simulink model "ModelNonLinear"  (R2014b)
settings: Solver=ode45  StartTime=0.0  StopTime=5  FixedStep=0.01  RelTol=1e-3
values from neighbouring files (symbols this model uses):
  H1 = -(R4*Rs/R1) * 1/(R7+Rv2)    [InitModel.m]    (also in SystemModel.m)
  R6 = 100e3    (= 100000)    [InitModel.m]    (also in SystemModel.m; SystemModel_marco.m)
  rad2rpm = 60/(2*pi)    (= 9.54929658551)    [InitModel.m]    (also in SystemModel.m)
  Vdc = 30    [InitModel.m]    (also in SystemModel.m; SystemModel_marco.m)
undefined symbols (not defined in the file or in its folder): motor, sigbuilder_block
libraries: cstblocks x5, simulink x1
settings Model: Creator=Edoardo  LastModifiedBy=Edoardo

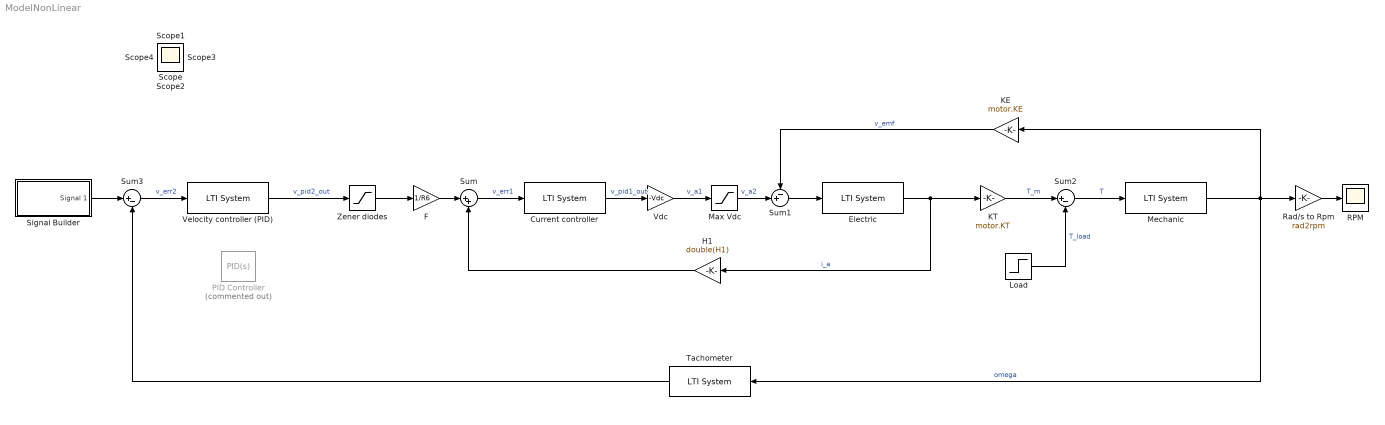
== system ModelNonLinear ==
  Current controller : cstblocks/LTI System  sys=C1  IC=[]
  Electric : cstblocks/LTI System  sys=G1  IC=[]
  F : Gain  Gain=1/R6
  H1 : Gain  Gain=double(H1)
  KE : Gain  Gain=motor.KE
  KT : Gain  Gain=motor.KT
  Load : Step  Time=2  After=0.02  SampleTime=0
  Max Vdc : Saturate  UpperLimit=30  LowerLimit=-30
  Mechanic : cstblocks/LTI System  sys=G2  IC=[]
  PID Controller : simulink/Continuous/PID Controller  Commented=on  Controller=PID  TimeDomain=Continuous-time  SampleTime=-1  IntegratorMethod=Forward Euler  FilterMethod=Forward Euler  Form=Parallel  P=9  I=18  D=0.001  N=100  InitialConditionSource=internal  InitialConditionForIntegrator=0  InitialConditionForFilter=0  ExternalReset=none  LimitOutput=off  UpperSaturationLimit=inf  LowerSaturationLimit=-inf  LinearizeAsGain=on  AntiWindupMode=none  Kb=1  TrackingMode=off  Kt=1  PParamMin=[]  PParamMax=[]  IParamMin=[]  IParamMax=[]  DParamMin=[]  DParamMax=[]  NParamMin=[]  NParamMax=[]  KbParamMin=[]  KbParamMax=[]  KtParamMin=[]  KtParamMax=[]  POutMin=[]  POutMax=[]  IOutMin=[]  IOutMax=[]  DOutMin=[]  DOutMax=[]  NOutMin=[]  NOutMax=[]  KbOutMin=[]  KbOutMax=[]  KtOutMin=[]  KtOutMax=[]  IntegratorOutMin=[]  IntegratorOutMax=[]  FilterOutMin=[]  FilterOutMax=[]  SumOutMin=[]  SumOutMax=[]  SumI1OutMin=[]  SumI1OutMax=[]  SumI2OutMin=[]  SumI2OutMax=[]  SumI3OutMin=[]  SumI3OutMax=[]  SumDOutMin=[]  SumDOutMax=[]  SaturationOutMin=[]  SaturationOutMax=[]  IntegratorContinuousStateAttributes=''  IntegratorStateMustResolveToSignalObject=off  IntegratorRTWStateStorageClass=Auto  FilterContinuousStateAttributes=''  FilterStateMustResolveToSignalObject=off  FilterRTWStateStorageClass=Auto  DifferentiatorICPrevScaledInput=0  DifferentiatorOutMin=[]  DifferentiatorOutMax=[]  UseFilter=on
  RPM : Scope
      settings: TimeRange=5  YMin=-1200  YMax=600  Decimation=100
  Rad/s to Rpm : Gain  Gain=rad2rpm
  Signal Builder : Subsystem  Tag=STV Subsys  LoadFcn=sigbuilder_block('load',[437.6 199.2 550.4 400 ]);  StartFcn=sigbuilder_block('start');  StopFcn=sigbuilder_block('stop');  ClipboardFcn=sigbuilder_block('clipboard');  mask(Sigbuilder block){}
      mask help: Simulink:masks:SigbuilderBlock_MD
      mask init:
      | if ~strcmp(get_param(bdroot(gcbh),'SimulationStatus'),'stopped') tuvar = sigbuilder_block('maskInit'); end
      settings: CopyFcn=sigbuilder_block('copy');  DeleteFcn=sigbuilder_block('delete');  ModelCloseFcn=sigbuilder_block('modelClose');  PreSaveFcn=sigbuilder_block('preSave');  PauseFcn=sigbuilder_block('pause');  ContinueFcn=sigbuilder_block('continue');  NameChangeFcn=sigbuilder_block('namechange');  OpenFcn=sigbuilder_block('open',[437.6 199.2 550.4 400 ]);  CloseFcn=sigbuilder_block('close');
      mask Display: plot(0, 0, 100, 100,[2, 2, 32, 32, 2], [68, 8, 8, 68, 68],[32, 2], [38, 38], [32, 19, 2],[53, 60, 44], [32, 17, 17, 2],[16, 16, 31, 31]);txt = getActiveGroup(gcbh);text(2, 100, txt,'verticalAlignment', 'top');
  Sum : Sum  Inputs=|++
  Sum1 : Sum  Inputs=-+|
  Sum2 : Sum  Inputs=|+-
  Sum3 : Sum  Inputs=|+-
  Tachometer : cstblocks/LTI System  sys=H2  IC=[]
  Vdc : Gain  Gain=-Vdc
  Velocity controller (PID) : cstblocks/LTI System  sys=C2  IC=[]
  Zener diodes : Saturate  UpperLimit=9  LowerLimit=-9
  Scope{,1..4} (5 alike) : Scope
      Scope settings: ShowLegends=on  YMin=0  YMax=0.15  SaveName=ScopeData5  Decimation=50
      Scope1 settings: YMin=0  YMax=1  Decimation=50
      Scope2 settings: ShowLegends=on  SaveName=ScopeData2  Decimation=10
      Scope3 settings: ShowLegends=on  YMin=0  YMax=12  SaveName=ScopeData3  Decimation=50
      Scope4 settings: ShowLegends=on  YMin=-0  YMax=25  SaveName=ScopeData4  Decimation=50
  wires:
  Sum1/1 -> Electric/1
  Current controller/1 -> Vdc/1  "v_pid1_out"
  Electric/1 -> H1/1, KT/1  "i_a"
  Mechanic/1 -> Tachometer/1, KE/1, Rad/s to Rpm/1  "omega"
  KT/1 -> Sum2/1  "T_m"
  Sum2/1 -> Mechanic/1  "T"
  Sum/1 -> Current controller/1  "v_err1"
  H1/1 -> Sum/2
  Sum3/1 -> Velocity controller (PID)/1  "v_err2"
  Tachometer/1 -> Sum3/2
  Rad/s to Rpm/1 -> RPM/1
  Signal Builder/1(Signal 1) -> Sum3/1
  Load/1 -> Sum2/2  "T_load"
  F/1 -> Sum/1
  Vdc/1 -> Max Vdc/1  "v_a1"
  Velocity controller (PID)/1 -> Zener diodes/1  "v_pid2_out"
  KE/1 -> Sum1/1  "v_emf"
  Zener diodes/1 -> F/1
  Max Vdc/1 -> Sum1/2  "v_a2"

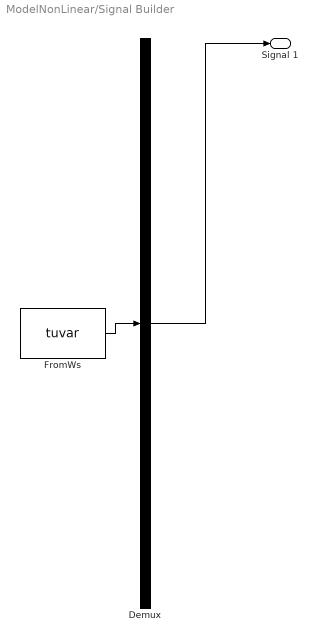
== system ModelNonLinear/Signal Builder ==
  Demux : Demux  Tag=STV Demux  Outputs=1
  FromWs : FromWorkspace  Tag=STV FromWs  VariableName=tuvar  SampleTime=0
      SigBuilderData=|
      | common.afterFinalStr = 'Extrapolate'
      | common.sampleTime = 0
      | dataSet.timeRange = [0 10]
      | dataSet.name = 'Group 1'
      | sbobj.Groups.Name = 'Group 1'
      | sbobj.Groups.Signals.Name = 'Signal 1'
      | sbobj.Groups.Signals.XData = [0 1 2 3 4 10]
      | sbobj.Groups.Signals.YData = [0 0 2 2 0 0]
  Signal 1 : Outport  Tag=STV Outport
  wires:
  Demux/1 -> Signal 1/1
  FromWs/1 -> Demux/1
